simulink model "modelOpt"  (Simulink 8.8)
settings: Solver=ode3  StartTime=0.0  StopTime=.4  FixedStep=.002  RelTol=1e-3  EnableMultiTasking=on
values from neighbouring files (symbols this model uses):
  A = 1    [plantParameters.m]
  B = B*a1    (= 0.058604)    [plantParameters.m]
  C = C*a2    (= 0.086832)    [plantParameters.m]
  heg = p(1)    [simMov.m]    (also in simulateHeadPerturbation.m = 1; simulateSubject.m = optimPar(i,1))
  stpc = head.time(trcHI{i,5}(2))    [optimization.m]    (also in simulateHeadPerturbation.m; simulateSubject.m)
  strc = head.time(trcHI{i,5}(1))    [optimization.m]    (also in simulateHeadPerturbation.m; simulateSubject.m)
  t1 = .224    (= 0.224)    [plantParameters.m]
  t2 = .013    (= 0.013)    [plantParameters.m]
  ts = tz    (= 0.08)    [plantParameters.m]
  vg = parHI(i,4)    [optimization.m]    (also in simulateHeadPerturbation.m = 0.3; simulateSubject.m)
  vs = p(2)    [simMov.m]    (also in simulateHeadPerturbation.m = optimPar(i,2); simulateSubject.m = optimPar(i,2))
  w = 200    [plantParameters.m]
  z = 1.2    [plantParameters.m]
settings Model: Creator=Paolo  LastModifiedBy=Paolo
settings DataIOCC: SignalLoggingSaveFormat=Dataset
settings DebuggingCC: SolverPrmCheckMsg=warning

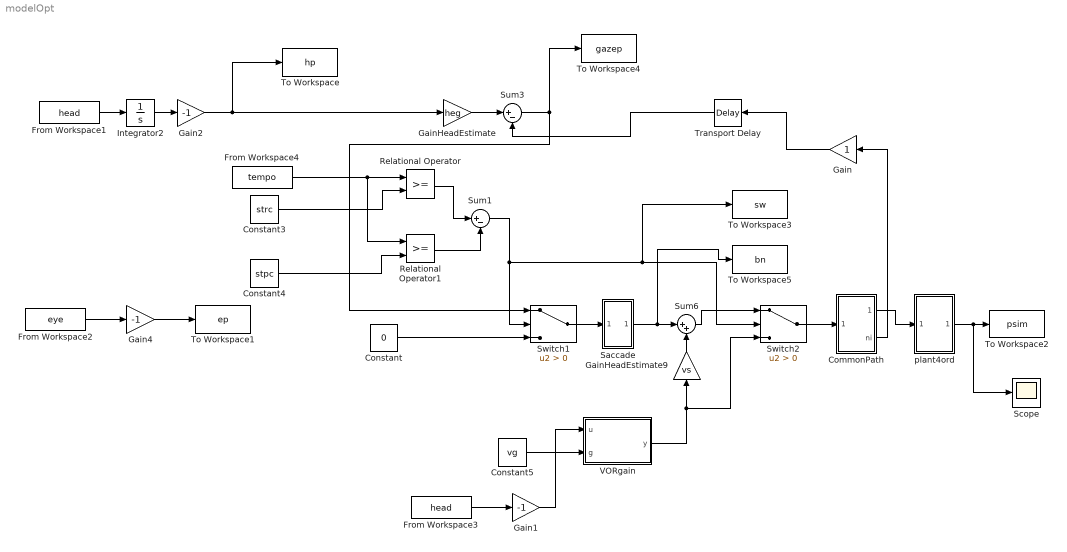
== system modelOpt ==
  CommonPath : Subsystem
  Constant : Constant  Value=0
  Constant3 : Constant  Value=strc
  Constant4 : Constant  Value=stpc
  Constant5 : Constant  Value=vg
  From Workspace1 : FromWorkspace  VariableName=head  SampleTime=0
  From Workspace2 : FromWorkspace  VariableName=eye  SampleTime=0
  From Workspace3 : FromWorkspace  VariableName=head  SampleTime=0
  From Workspace4 : FromWorkspace  VariableName=tempo  SampleTime=0
  Gain : Gain
  Gain1 : Gain  Gain=-1
  Gain2 : Gain  Gain=-1
  Gain4 : Gain  Gain=-1
  GainHeadEstimate : Gain  Gain=heg
  GainHeadEstimate9 : Gain  Gain=vs
  Integrator2 : Integrator
  Relational Operator : RelationalOperator  OutDataTypeStr=boolean  RndMeth=Nearest
  Relational Operator1 : RelationalOperator  OutDataTypeStr=boolean  RndMeth=Nearest
  Saccade : Subsystem
  Scope : Scope
  Sum1 : Sum  Inputs=|+-
  Sum3 : Sum  Inputs=|+-
  Sum6 : Sum  Inputs=|++
  Switch1 : Switch  Criteria=u2 > Threshold  ZeroCross=off
  Switch2 : Switch  Criteria=u2 > Threshold  ZeroCross=off
  To Workspace : ToWorkspace  VariableName=hp  SampleTime=-1
  To Workspace1 : ToWorkspace  VariableName=ep  SampleTime=-1
  To Workspace2 : ToWorkspace  VariableName=psim  SampleTime=-1
  To Workspace3 : ToWorkspace  VariableName=sw  SampleTime=-1
  To Workspace4 : ToWorkspace  VariableName=gazep  SampleTime=-1
  To Workspace5 : ToWorkspace  VariableName=bn  SampleTime=-1
  Transport Delay : TransportDelay  DelayTime=.006
  VORgain : MATLAB Function  TreatAsAtomicUnit=on
  plant4ord : Subsystem
  wires:
  CommonPath/1(cmd) -> plant4ord/1(In1)
  From Workspace3/1 -> Gain1/1
  Constant5/1 -> VORgain/2(g)
  Saccade/1(out_1) -> To Workspace5/1, Sum6/1
  GainHeadEstimate9/1 -> Sum6/2
  Switch1/1 -> Saccade/1(in_1)
  From Workspace1/1 -> Integrator2/1
  Gain2/1 -> To Workspace/1, GainHeadEstimate/1
  GainHeadEstimate/1 -> Sum3/1
  Sum3/1 -> To Workspace4/1, Switch1/1
  From Workspace2/1 -> Gain4/1
  Gain1/1 -> VORgain/1(u)
  Integrator2/1 -> Gain2/1
  Transport Delay/1 -> Sum3/2
  CommonPath/2(ni) -> Gain/1
  Gain/1 -> Transport Delay/1
  Gain4/1 -> To Workspace1/1
  plant4ord/1(Out1) -> Scope/1, To Workspace2/1
  Switch2/1 -> CommonPath/1(In1)
  VORgain/1(y) -> Switch2/3, GainHeadEstimate9/1
  From Workspace4/1 -> Relational Operator1/1, Relational Operator/1
  Constant3/1 -> Relational Operator/2
  Constant/1 -> Switch1/3
  Sum6/1 -> Switch2/1
  Constant4/1 -> Relational Operator1/2
  Relational Operator/1 -> Sum1/1
  Relational Operator1/1 -> Sum1/2
  Sum1/1 -> To Workspace3/1, Switch2/2, Switch1/2

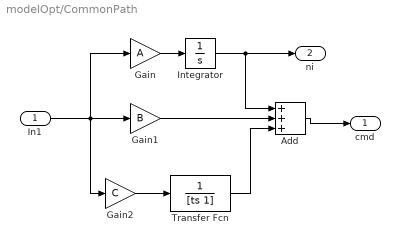
== system modelOpt/CommonPath ==
  In1 : Inport
  Add : Sum  Inputs=+++
  Gain : Gain  Gain=A
  Gain1 : Gain  Gain=B
  Gain2 : Gain  Gain=C
  Integrator : Integrator
  Transfer Fcn : TransferFcn  Denominator=[ts 1]
  cmd : Outport
  ni : Outport  Port=2
  wires:
  Gain/1 -> Integrator/1
  Gain2/1 -> Transfer Fcn/1
  In1/1 -> Gain/1, Gain1/1, Gain2/1
  Gain1/1 -> Add/2
  Integrator/1 -> Add/1, ni/1
  Transfer Fcn/1 -> Add/3
  Add/1 -> cmd/1

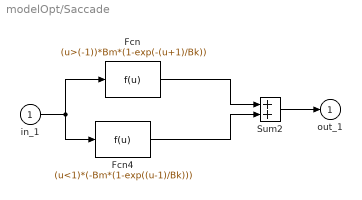
== system modelOpt/Saccade ==
  in_1 : Inport
  Fcn : Fcn  Expr=(u>(-1))*Bm*(1-exp(-(u+1)/Bk))
  Fcn4 : Fcn  Expr=(u<1)*(-Bm*(1-exp((u-1)/Bk)))
  Sum2 : Sum  SaturateOnIntegerOverflow=on  InputSameDT=on  OutDataTypeStr=Inherit: Same as first input
  out_1 : Outport  InitialOutput=0
  wires:
  Fcn4/1 -> Sum2/2
  Fcn/1 -> Sum2/1
  in_1/1 -> Fcn4/1, Fcn/1
  Sum2/1 -> out_1/1

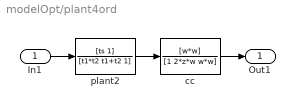
== system modelOpt/plant4ord ==
  In1 : Inport
  cc : TransferFcn  Numerator=[w*w]  Denominator=[1 2*z*w w*w]
  plant2 : TransferFcn  Numerator=[ts 1]  Denominator=[t1*t2 t1+t2 1]
  Out1 : Outport
  wires:
  plant2/1 -> cc/1
  In1/1 -> plant2/1
  cc/1 -> Out1/1

== matlab function VORgain ==
  data: u input double; y output double; g input double
function y = gain(u,g)
%#codegen
if u>0
    y=g*u;
else
    y=u;
end
